simulink model "SimulinkFullblock"  (R2019b)
settings: Solver=VariableStepAuto  StartTime=0.0  StopTime=10  RelTol=1e-3
(part 1 of 5)
settings Model: Creator=gasserelazab  LastModifiedBy=gasserelazab
settings DataIOCC: ReturnWorkspaceOutputs=off
settings DebuggingCC: ArithmeticOperatorsInVariantConditions=warning
settings SFSimCC: SimUseLocalCustomCode=off  CustomCodeUndefinedFunction=UseInterfaceOnly
settings RTWCC: RTWUseLocalCustomCode=off

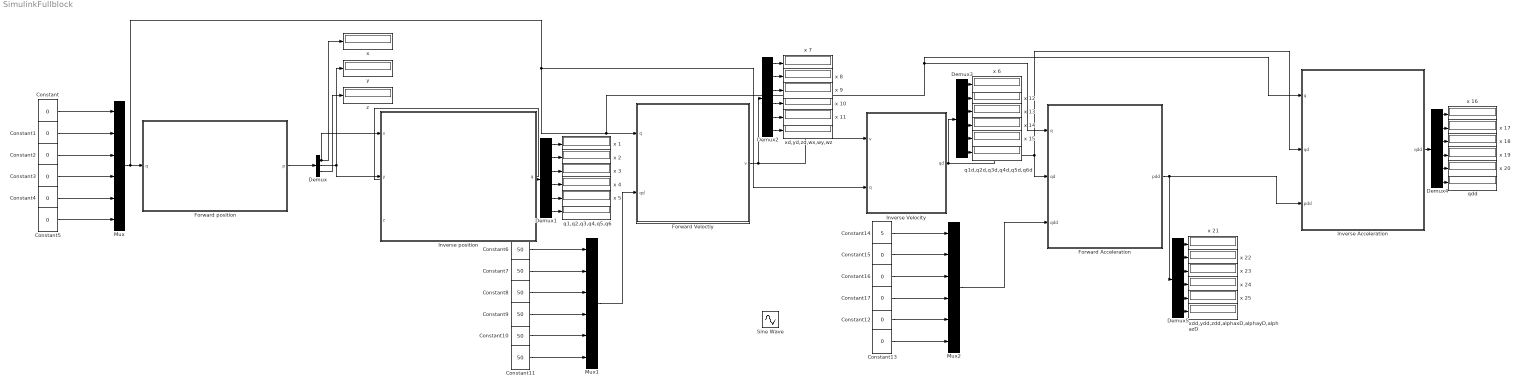
== system SimulinkFullblock ==
  " Inverse Velocity " : MATLAB Function  TreatAsAtomicUnit=on
  " xd,yd,zd,wx,wy,wz " : Display
  Constant{,1..5,12..13,15..17} (11 alike) : Constant  Value=0
  Constant{6..11} (6 alike) : Constant  Value=50
  Constant14 : Constant  Value=5
  Demux : Demux  Outputs=3
  Demux{1..5} (5 alike) : Demux  Outputs=6
  "Forward Acceleration " : MATLAB Function  TreatAsAtomicUnit=on
  Forward Veloctiy : MATLAB Function  TreatAsAtomicUnit=on
  "Forward position " : MATLAB Function  TreatAsAtomicUnit=on
  "Inverse Acceleration " : MATLAB Function  TreatAsAtomicUnit=on
  "Inverse position " : MATLAB Function  TreatAsAtomicUnit=on
  Mux : Mux  Inputs=6
  Mux1 : Mux  Inputs=6
  Mux2 : Mux  Inputs=6
  Sine Wave : Sin  SampleTime=0
  "q1,q2,q3,q4,q5,q6 " : Display
  "q1d,q2d,q3d,q4d,q5d,q6d " : Display
  "qdd " : Display
  x {,1..25} (26 alike) : Display
  "xdd,ydd,zdd,alphaxD,alphayD,alphazD " : Display
  y : Display
  z : Display
  wires:
  Mux/1 -> " Inverse Velocity "/2(q), "Inverse Acceleration "/1(q), "Forward Acceleration "/1(q), Forward Veloctiy/1(q), "Forward position "/1(q)
  Constant/1 -> Mux/1
  Constant1/1 -> Mux/2
  Constant2/1 -> Mux/3
  Constant3/1 -> Mux/4
  Constant4/1 -> Mux/5
  Constant5/1 -> Mux/6
  "Forward position "/1(p) -> Demux/1
  Demux/1 -> "Inverse position "/1(x), "x "/1
  Demux/2 -> "Inverse position "/2(y), y/1
  Demux/3 -> z/1
  "Inverse position "/1(q) -> Demux1/1
  Constant8/1 -> Mux1/3
  Constant6/1 -> Mux1/1
  Constant7/1 -> Mux1/2
  Mux1/1 -> Forward Veloctiy/2(qd)
  Constant9/1 -> Mux1/4
  Constant10/1 -> Mux1/5
  Constant11/1 -> Mux1/6
  Forward Veloctiy/1(v) -> Demux2/1, " Inverse Velocity "/1(v)
  " Inverse Velocity "/1(qd) -> Demux3/1, "Inverse Acceleration "/2(qd), "Forward Acceleration "/2(qd)
  Constant16/1 -> Mux2/3
  Constant13/1 -> Mux2/6
  Constant12/1 -> Mux2/5
  Constant15/1 -> Mux2/2
  Constant17/1 -> Mux2/4
  Mux2/1 -> "Forward Acceleration "/3(qdd)
  "Forward Acceleration "/1(pdd) -> Demux5/1, "Inverse Acceleration "/3(pdd)
  "Inverse Acceleration "/1(qdd) -> Demux4/1
  Demux1/2 -> x 2/1
  Demux1/1 -> x 1/1
  Demux1/3 -> x 3/1
  Demux1/4 -> x 4/1
  Demux1/5 -> x 5/1
  Demux1/6 -> "q1,q2,q3,q4,q5,q6 "/1
  Demux2/4 -> x 10/1
  Demux2/6 -> " xd,yd,zd,wx,wy,wz "/1
  Demux2/5 -> x 11/1
  Demux2/1 -> x 7/1
  Demux2/3 -> x 9/1
  Demux2/2 -> x 8/1
  Constant14/1 -> Mux2/1
  Demux3/5 -> x 15/1
  Demux3/4 -> x 14/1
  Demux3/6 -> "q1d,q2d,q3d,q4d,q5d,q6d "/1
  Demux3/3 -> x 13/1
  Demux3/2 -> x 12/1
  Demux3/1 -> x 6/1
  Demux4/1 -> x 16/1
  Demux4/2 -> x 17/1
  Demux4/3 -> x 18/1
  Demux4/4 -> x 19/1
  Demux4/5 -> x 20/1
  Demux4/6 -> "qdd "/1
  Demux5/6 -> "xdd,ydd,zdd,alphaxD,alphayD,alphazD "/1
  Demux5/2 -> x 22/1
  Demux5/5 -> x 25/1
  Demux5/1 -> x 21/1
  Demux5/4 -> x 24/1
  Demux5/3 -> x 23/1

== matlab function SimulinkFullblock/Inverse position  ==
  data: q output; x input; y input; z input
function q   = fcn(x, y, z)

qnew=[0;0;0;0;0;0];
qold=[50;50;50;50;50;50];

i=100;
dog=true;

while (i>0 && dog)
    q1=qold(1,1);
    q2=qold(2,1);
    q3=qold(3,1);
    q4=qold(4,1);
    q5=qold(5,1);
    q6=qold(6,1);
    
    F= [ 10*cos((pi*(q1 - 90))/180)*sin((pi*(q2 - 90))/180) - 10*sin((pi*(q5 + 90))/180)*(sin((pi*(q1 - 90))/180)*sin((pi*(q4 + 90))/180) - cos((pi*(q1 - 90))/180)*cos((pi*(q2 - 90))/180)*cos((pi*(q4 + 90))/180)) - x + cos((pi*(q1 - 90))/180)*sin((pi*(q2 - 90))/180)*(q3 + 10) - 10*cos((pi*(q1 - 90))/180)*cos((pi*(q5 + 90))/180)*sin((pi*(q2 - 90))/180);...
 10*sin((pi*(q5 + 90))/180)*(cos((pi*(q1 - 90))/180)*sin((pi*(q4 + 90))/180) + cos((pi*(q2 - 90))/180)*cos((pi*(q4 + 90))/180)*sin((pi*(q1 - 90))/180)) - y + 10*sin((pi*(q1 - 90))/180)*sin((pi*(q2 - 90))/180) + sin((pi*(q1 - 90))/180)*sin((pi*(q2 - 90))/180)*(q3 + 10) - 10*cos((pi*(q5 + 90))/180)*sin((pi*(q1 - 90))/180)*sin((pi*(q2 - 90))/180);...
                                                                                                                                                10*cos((pi*(q2 - 90))/180) - z + cos((pi*(q2 - 90))/180)*(q3 + 10) - 10*cos((pi*(q2 - 90))/180)*cos((pi*(q5 + 90))/180) - 10*cos((pi*(q4 + 90))/180)*sin((pi*(q2 - 90))/180)*sin((pi*(q5 + 90))/180) + 10];
 FJ= [ (pi*cos((pi*(q5 + 90))/180)*sin((pi*(q1 - 90))/180)*sin((pi*(q2 - 90))/180))/18 - (pi*sin((pi*(q1 - 90))/180)*sin((pi*(q2 - 90))/180))/18 - (pi*sin((pi*(q1 - 90))/180)*sin((pi*(q2 - 90))/180)*(q3 + 10))/180 - 10*sin((pi*(q5 + 90))/180)*((pi*cos((pi*(q1 - 90))/180)*sin((pi*(q4 + 90))/180))/180 + (pi*cos((pi*(q2 - 90))/180)*cos((pi*(q4 + 90))/180)*sin((pi*(q1 - 90))/180))/180), (pi*cos((pi*(q1 - 90))/180)*cos((pi*(q2 - 90))/180))/18 + (pi*cos((pi*(q1 - 90))/180)*cos((pi*(q2 - 90))/180)*(q3 + 10))/180 - (pi*cos((pi*(q1 - 90))/180)*cos((pi*(q2 - 90))/180)*cos((pi*(q5 + 90))/180))/18 - (pi*cos((pi*(q1 - 90))/180)*cos((pi*(q4 + 90))/180)*sin((pi*(q2 - 90))/180)*sin((pi*(q5 + 90))/180))/18, cos((pi*(q1 - 90))/180)*sin((pi*(q2 - 90))/180), -10*sin((pi*(q5 + 90))/180)*((pi*cos((pi*(q4 + 90))/180)*sin((pi*(q1 - 90))/180))/180 + (pi*cos((pi*(q1 - 90))/180)*cos((pi*(q2 - 90))/180)*sin((pi*(q4 + 90))/180))/180), (pi*cos((pi*(q1 - 90))/180)*sin((pi*(q2 - 90))/180)*sin((pi*(q5 + 90))/180))/18 - (pi*cos((pi*(q5 + 90))/180)*(sin((pi*(q1 - 90))/180)*sin((pi*(q4 + 90))/180) - cos((pi*(q1 - 90))/180)*cos((pi*(q2 - 90))/180)*cos((pi*(q4 + 90))/180)))/18, 0;...
 (pi*cos((pi*(q1 - 90))/180)*sin((pi*(q2 - 90))/180))/18 - 10*sin((pi*(q5 + 90))/180)*((pi*sin((pi*(q1 - 90))/180)*sin((pi*(q4 + 90))/180))/180 - (pi*cos((pi*(q1 - 90))/180)*cos((pi*(q2 - 90))/180)*cos((pi*(q4 + 90))/180))/180) + (pi*cos((pi*(q1 - 90))/180)*sin((pi*(q2 - 90))/180)*(q3 + 10))/180 - (pi*cos((pi*(q1 - 90))/180)*cos((pi*(q5 + 90))/180)*sin((pi*(q2 - 90))/180))/18, (pi*cos((pi*(q2 - 90))/180)*sin((pi*(q1 - 90))/180))/18 + (pi*cos((pi*(q2 - 90))/180)*sin((pi*(q1 - 90))/180)*(q3 + 10))/180 - (pi*cos((pi*(q2 - 90))/180)*cos((pi*(q5 + 90))/180)*sin((pi*(q1 - 90))/180))/18 - (pi*cos((pi*(q4 + 90))/180)*sin((pi*(q1 - 90))/180)*sin((pi*(q2 - 90))/180)*sin((pi*(q5 + 90))/180))/18, sin((pi*(q1 - 90))/180)*sin((pi*(q2 - 90))/180),  10*sin((pi*(q5 + 90))/180)*((pi*cos((pi*(q1 - 90))/180)*cos((pi*(q4 + 90))/180))/180 - (pi*cos((pi*(q2 - 90))/180)*sin((pi*(q1 - 90))/180)*sin((pi*(q4 + 90))/180))/180), (pi*cos((pi*(q5 + 90))/180)*(cos((pi*(q1 - 90))/180)*sin((pi*(q4 + 90))/180) + cos((pi*(q2 - 90))/180)*cos((pi*(q4 + 90))/180)*sin((pi*(q1 - 90))/180)))/18 + (pi*sin((pi*(q1 - 90))/180)*sin((pi*(q2 - 90))/180)*sin((pi*(q5 + 90))/180))/18, 0;...
                                                                                                                                                                                                                                                                                                                                                                                         0,                                                                                                 (pi*cos((pi*(q5 + 90))/180)*sin((pi*(q2 - 90))/180))/18 - (pi*sin((pi*(q2 - 90))/180)*(q3 + 10))/180 - (pi*sin((pi*(q2 - 90))/180))/18 - (pi*cos((pi*(q2 - 90))/180)*cos((pi*(q4 + 90))/180)*sin((pi*(q5 + 90))/180))/18,                         cos((pi*(q2 - 90))/180),                                                                                           (pi*sin((pi*(q2 - 90))/180)*sin((pi*(q4 + 90))/180)*sin((pi*(q5 + 90))/180))/18,                                                                                                     (pi*cos((pi*(q2 - 90))/180)*sin((pi*(q5 + 90))/180))/18 - (pi*cos((pi*(q4 + 90))/180)*cos((pi*(q5 + 90))/180)*sin((pi*(q2 - 90))/180))/18, 0];
 

    inverseFJ= transpose(FJ)*(inv(FJ*transpose(FJ)));
        
 
    qnew=qold-inverseFJ*F;
    %disp(inverseFJ*F);
    
  
   
    count=0;
   
   	for xx = 1:6
        if  ((qnew(xx,1)-qold(xx,1)<0.1) && (qnew(xx,1)-qold(xx,1)>-0.1 ))       
             count=count+1;
         end
   
    end
    
    if( count == 6)
        dog=false;
    end
    
    i=i-1;
    
    %disp(i);
    
    qold=qnew;
    
end
q=qold;

== matlab function SimulinkFullblock/Forward position  ==
  data: p output; q input
function p  = fcn(q)
q1= q(1);
q2= q(2);
q3= q(3);
q4= q(4);
q5= q(5);
q6= q(6);
L1=10;
L2=10;
L3=10;
L4=10;
pp= [ sin((pi*q6)/180)*(cos((pi*(q4 + 90))/180)*sin((pi*(q1 - 90))/180) + cos((pi*(q1 - 90))/180)*cos((pi*(q2 - 90))/180)*sin((pi*(q4 + 90))/180)) - cos((pi*q6)/180)*(cos((pi*(q5 + 90))/180)*(sin((pi*(q1 - 90))/180)*sin((pi*(q4 + 90))/180) - cos((pi*(q1 - 90))/180)*cos((pi*(q2 - 90))/180)*cos((pi*(q4 + 90))/180)) - cos((pi*(q1 - 90))/180)*sin((pi*(q2 - 90))/180)*sin((pi*(q5 + 90))/180)),   sin((pi*q6)/180)*(cos((pi*(q5 + 90))/180)*(sin((pi*(q1 - 90))/180)*sin((pi*(q4 + 90))/180) - cos((pi*(q1 - 90))/180)*cos((pi*(q2 - 90))/180)*cos((pi*(q4 + 90))/180)) - cos((pi*(q1 - 90))/180)*sin((pi*(q2 - 90))/180)*sin((pi*(q5 + 90))/180)) + cos((pi*q6)/180)*(cos((pi*(q4 + 90))/180)*sin((pi*(q1 - 90))/180) + cos((pi*(q1 - 90))/180)*cos((pi*(q2 - 90))/180)*sin((pi*(q4 + 90))/180)), - sin((pi*(q5 + 90))/180)*(sin((pi*(q1 - 90))/180)*sin((pi*(q4 + 90))/180) - cos((pi*(q1 - 90))/180)*cos((pi*(q2 - 90))/180)*cos((pi*(q4 + 90))/180)) - cos((pi*(q1 - 90))/180)*cos((pi*(q5 + 90))/180)*sin((pi*(q2 - 90))/180), cos((pi*(q1 - 90))/180)*sin((pi*(q2 - 90))/180)*(L2 + q3) - L4*(sin((pi*(q5 + 90))/180)*(sin((pi*(q1 - 90))/180)*sin((pi*(q4 + 90))/180) - cos((pi*(q1 - 90))/180)*cos((pi*(q2 - 90))/180)*cos((pi*(q4 + 90))/180)) + cos((pi*(q1 - 90))/180)*cos((pi*(q5 + 90))/180)*sin((pi*(q2 - 90))/180)) + L3*cos((pi*(q1 - 90))/180)*sin((pi*(q2 - 90))/180);
 cos((pi*q6)/180)*(cos((pi*(q5 + 90))/180)*(cos((pi*(q1 - 90))/180)*sin((pi*(q4 + 90))/180) + cos((pi*(q2 - 90))/180)*cos((pi*(q4 + 90))/180)*sin((pi*(q1 - 90))/180)) + sin((pi*(q1 - 90))/180)*sin((pi*(q2 - 90))/180)*sin((pi*(q5 + 90))/180)) - sin((pi*q6)/180)*(cos((pi*(q1 - 90))/180)*cos((pi*(q4 + 90))/180) - cos((pi*(q2 - 90))/180)*sin((pi*(q1 - 90))/180)*sin((pi*(q4 + 90))/180)), - sin((pi*q6)/180)*(cos((pi*(q5 + 90))/180)*(cos((pi*(q1 - 90))/180)*sin((pi*(q4 + 90))/180) + cos((pi*(q2 - 90))/180)*cos((pi*(q4 + 90))/180)*sin((pi*(q1 - 90))/180)) + sin((pi*(q1 - 90))/180)*sin((pi*(q2 - 90))/180)*sin((pi*(q5 + 90))/180)) - cos((pi*q6)/180)*(cos((pi*(q1 - 90))/180)*cos((pi*(q4 + 90))/180) - cos((pi*(q2 - 90))/180)*sin((pi*(q1 - 90))/180)*sin((pi*(q4 + 90))/180)),   sin((pi*(q5 + 90))/180)*(cos((pi*(q1 - 90))/180)*sin((pi*(q4 + 90))/180) + cos((pi*(q2 - 90))/180)*cos((pi*(q4 + 90))/180)*sin((pi*(q1 - 90))/180)) - cos((pi*(q5 + 90))/180)*sin((pi*(q1 - 90))/180)*sin((pi*(q2 - 90))/180), L4*(sin((pi*(q5 + 90))/180)*(cos((pi*(q1 - 90))/180)*sin((pi*(q4 + 90))/180) + cos((pi*(q2 - 90))/180)*cos((pi*(q4 + 90))/180)*sin((pi*(q1 - 90))/180)) - cos((pi*(q5 + 90))/180)*sin((pi*(q1 - 90))/180)*sin((pi*(q2 - 90))/180)) + sin((pi*(q1 - 90))/180)*sin((pi*(q2 - 90))/180)*(L2 + q3) + L3*sin((pi*(q1 - 90))/180)*sin((pi*(q2 - 90))/180);
                                                                                                                                                                                 cos((pi*q6)/180)*(cos((pi*(q2 - 90))/180)*sin((pi*(q5 + 90))/180) - cos((pi*(q4 + 90))/180)*cos((pi*(q5 + 90))/180)*sin((pi*(q2 - 90))/180)) - sin((pi*q6)/180)*sin((pi*(q2 - 90))/180)*sin((pi*(q4 + 90))/180),                                                                                                                                                                                 - sin((pi*q6)/180)*(cos((pi*(q2 - 90))/180)*sin((pi*(q5 + 90))/180) - cos((pi*(q4 + 90))/180)*cos((pi*(q5 + 90))/180)*sin((pi*(q2 - 90))/180)) - cos((pi*q6)/180)*sin((pi*(q2 - 90))/180)*sin((pi*(q4 + 90))/180),                                                                                                     - cos((pi*(q2 - 90))/180)*cos((pi*(q5 + 90))/180) - cos((pi*(q4 + 90))/180)*sin((pi*(q2 - 90))/180)*sin((pi*(q5 + 90))/180),                                                                                                                                                L1 - L4*(cos((pi*(q2 - 90))/180)*cos((pi*(q5 + 90))/180) + cos((pi*(q4 + 90))/180)*sin((pi*(q2 - 90))/180)*sin((pi*(q5 + 90))/180)) + cos((pi*(q2 - 90))/180)*(L2 + q3) + L3*cos((pi*(q2 - 90))/180);
                                                                                                                                                                                                                                                                                                                                                                                               0,                                                                                                                                                                                                                                                                                                                                                                                                 0,                                                                                                                                                                                                                               0,                                                                                                                                                                                                                                                                                                                                                   1];
x=pp(1,4);
y=pp(2,4);
z=pp(3,4);
p= [x;y;z];

== matlab function SimulinkFullblock/Forward Veloctiy ==
  data: q input; v output; qd input
function v   = fcn(q,qd)
q1= q(1);
q2= q(2);
q3= q(3);
q4= q(4);
q5= q(5);
q6= q(6);
q1d=qd(1);
q2d=qd(2);
q3d=qd(3);
q4d=qd(4);
q5d=qd(5);
q6d=qd(6);
L1=10;
L2=10;
L3=10;
L4=10;

A0T1= [ cos(0.0175*q1 - 1.5708),  0, -sin(0.0175*q1 - 1.5708),  0;...
 sin(0.0175*q1 - 1.5708),  0,  cos(0.0175*q1 - 1.5708),  0;...
                       0, -1,                        0, L1];
                   


A0T2= [ cos(0.0175*q1 - 1.5708)*cos(0.0175*q2 - 1.5708), -sin(0.0175*q1 - 1.5708), cos(0.0175*q1 - 1.5708)*sin(0.0175*q2 - 1.5708),  0;...
 cos(0.0175*q2 - 1.5708)*sin(0.0175*q1 - 1.5708),  cos(0.0175*q1 - 1.5708), sin(0.0175*q1 - 1.5708)*sin(0.0175*q2 - 1.5708),  0;...
                        -sin(0.0175*q2 - 1.5708),                        0,                         cos(0.0175*q2 - 1.5708), L1];
                                        
A0T3=  [ cos(0.0175*q1 - 1.5708)*cos(0.0175*q2 - 1.5708), -sin(0.0175*q1 - 1.5708), cos(0.0175*q1 - 1.5708)*sin(0.0175*q2 - 1.5708), cos(0.0175*q1 - 1.5708)*sin(0.0175*q2 - 1.5708)*(L2 + q3);...
 cos(0.0175*q2 - 1.5708)*sin(0.0175*q1 - 1.5708),  cos(0.0175*q1 - 1.5708), sin(0.0175*q1 - 1.5708)*sin(0.0175*q2 - 1.5708), sin(0.0175*q1 - 1.5708)*sin(0.0175*q2 - 1.5708)*(L2 + q3);...
                        -sin(0.0175*q2 - 1.5708),                        0,                         cos(0.0175*q2 - 1.5708),                    L1 + cos(0.0175*q2 - 1.5708)*(L2 + q3)];
                    
A0T4= [ cos(0.0175*q1 - 1.5708)*cos(0.0175*q2 - 1.5708)*cos(0.0175*q4 + 1.5708) - sin(0.0175*q1 - 1.5708)*sin(0.0175*q4 + 1.5708), cos(0.0175*q1 - 1.5708)*sin(0.0175*q2 - 1.5708), cos(0.0175*q4 + 1.5708)*sin(0.0175*q1 - 1.5708) + cos(0.0175*q1 - 1.5708)*cos(0.0175*q2 - 1.5708)*sin(0.0175*q4 + 1.5708), cos(0.0175*q1 - 1.5708)*sin(0.0175*q2 - 1.5708)*(L2 + q3) + L3*cos(0.0175*q1 - 1.5708)*sin(0.0175*q2 - 1.5708);...
 cos(0.0175*q1 - 1.5708)*sin(0.0175*q4 + 1.5708) + cos(0.0175*q2 - 1.5708)*cos(0.0175*q4 + 1.5708)*sin(0.0175*q1 - 1.5708), sin(0.0175*q1 - 1.5708)*sin(0.0175*q2 - 1.5708), cos(0.0175*q2 - 1.5708)*sin(0.0175*q1 - 1.5708)*sin(0.0175*q4 + 1.5708) - cos(0.0175*q1 - 1.5708)*cos(0.0175*q4 + 1.5708), sin(0.0175*q1 - 1.5708)*sin(0.0175*q2 - 1.5708)*(L2 + q3) + L3*sin(0.0175*q1 - 1.5708)*sin(0.0175*q2 - 1.5708);...
                                                                          -cos(0.0175*q4 + 1.5708)*sin(0.0175*q2 - 1.5708),                         cos(0.0175*q2 - 1.5708),                                                                          -sin(0.0175*q2 - 1.5708)*sin(0.0175*q4 + 1.5708),                                            L1 + cos(0.0175*q2 - 1.5708)*(L2 + q3) + L3*cos(0.0175*q2 - 1.5708)];
                                                                      
A0T5= [ cos(0.0175*q1 - 1.5708)*sin(0.0175*q2 - 1.5708)*sin(0.0175*q5 + 1.5708) - cos(0.0175*q5 + 1.5708)*(sin(0.0175*q1 - 1.5708)*sin(0.0175*q4 + 1.5708) - cos(0.0175*q1 - 1.5708)*cos(0.0175*q2 - 1.5708)*cos(0.0175*q4 + 1.5708)), cos(0.0175*q4 + 1.5708)*sin(0.0175*q1 - 1.5708) + cos(0.0175*q1 - 1.5708)*cos(0.0175*q2 - 1.5708)*sin(0.0175*q4 + 1.5708), - sin(0.0175*q5 + 1.5708)*(sin(0.0175*q1 - 1.5708)*sin(0.0175*q4 + 1.5708) - cos(0.0175*q1 - 1.5708)*cos(0.0175*q2 - 1.5708)*cos(0.0175*q4 + 1.5708)) - cos(0.0175*q1 - 1.5708)*cos(0.0175*q5 + 1.5708)*sin(0.0175*q2 - 1.5708), cos(0.0175*q1 - 1.5708)*sin(0.0175*q2 - 1.5708)*(L2 + q3) + L3*cos(0.0175*q1 - 1.5708)*sin(0.0175*q2 - 1.5708);...
 cos(0.0175*q5 + 1.5708)*(cos(0.0175*q1 - 1.5708)*sin(0.0175*q4 + 1.5708) + cos(0.0175*q2 - 1.5708)*cos(0.0175*q4 + 1.5708)*sin(0.0175*q1 - 1.5708)) + sin(0.0175*q1 - 1.5708)*sin(0.0175*q2 - 1.5708)*sin(0.0175*q5 + 1.5708), cos(0.0175*q2 - 1.5708)*sin(0.0175*q1 - 1.5708)*sin(0.0175*q4 + 1.5708) - cos(0.0175*q1 - 1.5708)*cos(0.0175*q4 + 1.5708),   sin(0.0175*q5 + 1.5708)*(cos(0.0175*q1 - 1.5708)*sin(0.0175*q4 + 1.5708) + cos(0.0175*q2 - 1.5708)*cos(0.0175*q4 + 1.5708)*sin(0.0175*q1 - 1.5708)) - cos(0.0175*q5 + 1.5708)*sin(0.0175*q1 - 1.5708)*sin(0.0175*q2 - 1.5708), sin(0.0175*q1 - 1.5708)*sin(0.0175*q2 - 1.5708)*(L2 + q3) + L3*sin(0.0175*q1 - 1.5708)*sin(0.0175*q2 - 1.5708);...
                                                                                                     cos(0.0175*q2 - 1.5708)*sin(0.0175*q5 + 1.5708) - cos(0.0175*q4 + 1.5708)*cos(0.0175*q5 + 1.5708)*sin(0.0175*q2 - 1.5708),                                                                          -sin(0.0175*q2 - 1.5708)*sin(0.0175*q4 + 1.5708),                                                                                                     - cos(0.0175*q2 - 1.5708)*cos(0.0175*q5 + 1.5708) - cos(0.0175*q4 + 1.5708)*sin(0.0175*q2 - 1.5708)*sin(0.0175*q5 + 1.5708),                                            L1 + cos(0.0175*q2 - 1.5708)*(L2 + q3) + L3*cos(0.0175*q2 - 1.5708)];
                                                                                                 
                                                                                                 
A0T6= [ sin((pi*q6)/180)*(cos((pi*(q4 + 90))/180)*sin((pi*(q1 - 90))/180) + cos((pi*(q1 - 90))/180)*cos((pi*(q2 - 90))/180)*sin((pi*(q4 + 90))/180)) - cos((pi*q6)/180)*(cos((pi*(q5 + 90))/180)*(sin((pi*(q1 - 90))/180)*sin((pi*(q4 + 90))/180) - cos((pi*(q1 - 90))/180)*cos((pi*(q2 - 90))/180)*cos((pi*(q4 + 90))/180)) - cos((pi*(q1 - 90))/180)*sin((pi*(q2 - 90))/180)*sin((pi*(q5 + 90))/180)),   sin((pi*q6)/180)*(cos((pi*(q5 + 90))/180)*(sin((pi*(q1 - 90))/180)*sin((pi*(q4 + 90))/180) - cos((pi*(q1 - 90))/180)*cos((pi*(q2 - 90))/180)*cos((pi*(q4 + 90))/180)) - cos((pi*(q1 - 90))/180)*sin((pi*(q2 - 90))/180)*sin((pi*(q5 + 90))/180)) + cos((pi*q6)/180)*(cos((pi*(q4 + 90))/180)*sin((pi*(q1 - 90))/180) + cos((pi*(q1 - 90))/180)*cos((pi*(q2 - 90))/180)*sin((pi*(q4 + 90))/180)), - sin((pi*(q5 + 90))/180)*(sin((pi*(q1 - 90))/180)*sin((pi*(q4 + 90))/180) - cos((pi*(q1 - 90))/180)*cos((pi*(q2 - 90))/180)*cos((pi*(q4 + 90))/180)) - cos((pi*(q1 - 90))/180)*cos((pi*(q5 + 90))/180)*sin((pi*(q2 - 90))/180), cos((pi*(q1 - 90))/180)*sin((pi*(q2 - 90))/180)*(L2 + q3) - L4*(sin((pi*(q5 + 90))/180)*(sin((pi*(q1 - 90))/180)*sin((pi*(q4 + 90))/180) - cos((pi*(q1 - 90))/180)*cos((pi*(q2 - 90))/180)*cos((pi*(q4 + 90))/180)) + cos((pi*(q1 - 90))/180)*cos((pi*(q5 + 90))/180)*sin((pi*(q2 - 90))/180)) + L3*cos((pi*(q1 - 90))/180)*sin((pi*(q2 - 90))/180);
 cos((pi*q6)/180)*(cos((pi*(q5 + 90))/180)*(cos((pi*(q1 - 90))/180)*sin((pi*(q4 + 90))/180) + cos((pi*(q2 - 90))/180)*cos((pi*(q4 + 90))/180)*sin((pi*(q1 - 90))/180)) + sin((pi*(q1 - 90))/180)*sin((pi*(q2 - 90))/180)*sin((pi*(q5 + 90))/180)) - sin((pi*q6)/180)*(cos((pi*(q1 - 90))/180)*cos((pi*(q4 + 90))/180) - cos((pi*(q2 - 90))/180)*sin((pi*(q1 - 90))/180)*sin((pi*(q4 + 90))/180)), - sin((pi*q6)/180)*(cos((pi*(q5 + 90))/180)*(cos((pi*(q1 - 90))/180)*sin((pi*(q4 + 90))/180) + cos((pi*(q2 - 90))/180)*cos((pi*(q4 + 90))/180)*sin((pi*(q1 - 90))/180)) + sin((pi*(q1 - 90))/180)*sin((pi*(q2 - 90))/180)*sin((pi*(q5 + 90))/180)) - cos((pi*q6)/180)*(cos((pi*(q1 - 90))/180)*cos((pi*(q4 + 90))/180) - cos((pi*(q2 - 90))/180)*sin((pi*(q1 - 90))/180)*sin((pi*(q4 + 90))/180)),   sin((pi*(q5 + 90))/180)*(cos((pi*(q1 - 90))/180)*sin((pi*(q4 + 90))/180) + cos((pi*(q2 - 90))/180)*cos((pi*(q4 + 90))/180)*sin((pi*(q1 - 90))/180)) - cos((pi*(q5 + 90))/180)*sin((pi*(q1 - 90))/180)*sin((pi*(q2 - 90))/180), L4*(sin((pi*(q5 + 90))/180)*(cos((pi*(q1 - 90))/180)*sin((pi*(q4 + 90))/180) + cos((pi*(q2 - 90))/180)*cos((pi*(q4 + 90))/180)*sin((pi*(q1 - 90))/180)) - cos((pi*(q5 + 90))/180)*sin((pi*(q1 - 90))/180)*sin((pi*(q2 - 90))/180)) + sin((pi*(q1 - 90))/180)*sin((pi*(q2 - 90))/180)*(L2 + q3) + L3*sin((pi*(q1 - 90))/180)*sin((pi*(q2 - 90))/180);
                                                                                                                                                                                 cos((pi*q6)/180)*(cos((pi*(q2 - 90))/180)*sin((pi*(q5 + 90))/180) - cos((pi*(q4 + 90))/180)*cos((pi*(q5 + 90))/180)*sin((pi*(q2 - 90))/180)) - sin((pi*q6)/180)*sin((pi*(q2 - 90))/180)*sin((pi*(q4 + 90))/180),                                                                                                                                                                                 - sin((pi*q6)/180)*(cos((pi*(q2 - 90))/180)*sin((pi*(q5 + 90))/180) - cos((pi*(q4 + 90))/180)*cos((pi*(q5 + 90))/180)*sin((pi*(q2 - 90))/180)) - cos((pi*q6)/180)*sin((pi*(q2 - 90))/180)*sin((pi*(q4 + 90))/180),                                                                                                     - cos((pi*(q2 - 90))/180)*cos((pi*(q5 + 90))/180) - cos((pi*(q4 + 90))/180)*sin((pi*(q2 - 90))/180)*sin((pi*(q5 + 90))/180),                                                                                                                                                L1 - L4*(cos((pi*(q2 - 90))/180)*cos((pi*(q5 + 90))/180) + cos((pi*(q4 + 90))/180)*sin((pi*(q2 - 90))/180)*sin((pi*(q5 + 90))/180)) + cos((pi*(q2 - 90))/180)*(L2 + q3) + L3*cos((pi*(q2 - 90))/180)];
                                                                                                                                                                                                                                  
                                                                                                                   
 
Jv1= cross([0;0;1], A0T6(:,4)-[0;0;0]); 
Jv2= cross(A0T1(:,3),(A0T6(:,4)-A0T1(:,4)));
Jv3= A0T3(:,3);
Jv4= cross(A0T3(:,3),(A0T6(:,4)-A0T3(:,4)));
Jv5= cross(A0T4(:,3),(A0T6(:,4)-A0T4(:,4)));
Jv6= cross(A0T5(:,3),(A0T6(:,4)-A0T5(:,4)));

Jw1=[0;0;1];
Jw2= A0T1(:,3);
Jw3=[0;0;0];
Jw4= A0T3(:,3);
Jw5= A0T4(:,3);
Jw6= A0T5(:,3);
v= [Jv1 Jv2 Jv3 Jv4 Jv5 Jv6; Jw1 Jw2 Jw3 Jw4 Jw5 Jw6]*[q1d;q2d;q3d;q4d;q5d;q6d];

== matlab function SimulinkFullblock/ Inverse Velocity  ==
  data: v input; qd output; q input
function qd  = fcn(v,q)
xd=v(1);
yd=v(2);
zd=v(3);
wx=v(4);
wy=v(5);
wz=v(6);
q1= q(1);
q2= q(2);
q3= q(3);
q4= q(4);
q5= q(5);
q6= q(6);
L1=10;
L2=10;
L3=10;
L4=10;

A0T1= [ cos(0.0175*q1 - 1.5708),  0, -sin(0.0175*q1 - 1.5708),  0;...
 sin(0.0175*q1 - 1.5708),  0,  cos(0.0175*q1 - 1.5708),  0;...
                       0, -1,                        0, L1];
                   


A0T2= [ cos(0.0175*q1 - 1.5708)*cos(0.0175*q2 - 1.5708), -sin(0.0175*q1 - 1.5708), cos(0.0175*q1 - 1.5708)*sin(0.0175*q2 - 1.5708),  0;...
 cos(0.0175*q2 - 1.5708)*sin(0.0175*q1 - 1.5708),  cos(0.0175*q1 - 1.5708), sin(0.0175*q1 - 1.5708)*sin(0.0175*q2 - 1.5708),  0;...
                        -sin(0.0175*q2 - 1.5708),                        0,                         cos(0.0175*q2 - 1.5708), L1];
                                        
A0T3=  [ cos(0.0175*q1 - 1.5708)*cos(0.0175*q2 - 1.5708), -sin(0.0175*q1 - 1.5708), cos(0.0175*q1 - 1.5708)*sin(0.0175*q2 - 1.5708), cos(0.0175*q1 - 1.5708)*sin(0.0175*q2 - 1.5708)*(L2 + q3);...
 cos(0.0175*q2 - 1.5708)*sin(0.0175*q1 - 1.5708),  cos(0.0175*q1 - 1.5708), sin(0.0175*q1 - 1.5708)*sin(0.0175*q2 - 1.5708), sin(0.0175*q1 - 1.5708)*sin(0.0175*q2 - 1.5708)*(L2 + q3);...
                        -sin(0.0175*q2 - 1.5708),                        0,                         cos(0.0175*q2 - 1.5708),                    L1 + cos(0.0175*q2 - 1.5708)*(L2 + q3)];
                    
A0T4= [ cos(0.0175*q1 - 1.5708)*cos(0.0175*q2 - 1.5708)*cos(0.0175*q4 + 1.5708) - sin(0.0175*q1 - 1.5708)*sin(0.0175*q4 + 1.5708), cos(0.0175*q1 - 1.5708)*sin(0.0175*q2 - 1.5708), cos(0.0175*q4 + 1.5708)*sin(0.0175*q1 - 1.5708) + cos(0.0175*q1 - 1.5708)*cos(0.0175*q2 - 1.5708)*sin(0.0175*q4 + 1.5708), cos(0.0175*q1 - 1.5708)*sin(0.0175*q2 - 1.5708)*(L2 + q3) + L3*cos(0.0175*q1 - 1.5708)*sin(0.0175*q2 - 1.5708);...
 cos(0.0175*q1 - 1.5708)*sin(0.0175*q4 + 1.5708) + cos(0.0175*q2 - 1.5708)*cos(0.0175*q4 + 1.5708)*sin(0.0175*q1 - 1.5708), sin(0.0175*q1 - 1.5708)*sin(0.0175*q2 - 1.5708), cos(0.0175*q2 - 1.5708)*sin(0.0175*q1 - 1.5708)*sin(0.0175*q4 + 1.5708) - cos(0.0175*q1 - 1.5708)*cos(0.0175*q4 + 1.5708), sin(0.0175*q1 - 1.5708)*sin(0.0175*q2 - 1.5708)*(L2 + q3) + L3*sin(0.0175*q1 - 1.5708)*sin(0.0175*q2 - 1.5708);...
                                                                          -cos(0.0175*q4 + 1.5708)*sin(0.0175*q2 - 1.5708),                         cos(0.0175*q2 - 1.5708),                                                                          -sin(0.0175*q2 - 1.5708)*sin(0.0175*q4 + 1.5708),                                            L1 + cos(0.0175*q2 - 1.5708)*(L2 + q3) + L3*cos(0.0175*q2 - 1.5708)];
                                                                      
A0T5= [ cos(0.0175*q1 - 1.5708)*sin(0.0175*q2 - 1.5708)*sin(0.0175*q5 + 1.5708) - cos(0.0175*q5 + 1.5708)*(sin(0.0175*q1 - 1.5708)*sin(0.0175*q4 + 1.5708) - cos(0.0175*q1 - 1.5708)*cos(0.0175*q2 - 1.5708)*cos(0.0175*q4 + 1.5708)), cos(0.0175*q4 + 1.5708)*sin(0.0175*q1 - 1.5708) + cos(0.0175*q1 - 1.5708)*cos(0.0175*q2 - 1.5708)*sin(0.0175*q4 + 1.5708), - sin(0.0175*q5 + 1.5708)*(sin(0.0175*q1 - 1.5708)*sin(0.0175*q4 + 1.5708) - cos(0.0175*q1 - 1.5708)*cos(0.0175*q2 - 1.5708)*cos(0.0175*q4 + 1.5708)) - cos(0.0175*q1 - 1.5708)*cos(0.0175*q5 + 1.5708)*sin(0.0175*q2 - 1.5708), cos(0.0175*q1 - 1.5708)*sin(0.0175*q2 - 1.5708)*(L2 + q3) + L3*cos(0.0175*q1 - 1.5708)*sin(0.0175*q2 - 1.5708);...
 cos(0.0175*q5 + 1.5708)*(cos(0.0175*q1 - 1.5708)*sin(0.0175*q4 + 1.5708) + cos(0.0175*q2 - 1.5708)*cos(0.0175*q4 + 1.5708)*sin(0.0175*q1 - 1.5708)) + sin(0.0175*q1 - 1.5708)*sin(0.0175*q2 - 1.5708)*sin(0.0175*q5 + 1.5708), cos(0.0175*q2 - 1.5708)*sin(0.0175*q1 - 1.5708)*sin(0.0175*q4 + 1.5708) - cos(0.0175*q1 - 1.5708)*cos(0.0175*q4 + 1.5708),   sin(0.0175*q5 + 1.5708)*(cos(0.0175*q1 - 1.5708)*sin(0.0175*q4 + 1.5708) + cos(0.0175*q2 - 1.5708)*cos(0.0175*q4 + 1.5708)*sin(0.0175*q1 - 1.5708)) - cos(0.0175*q5 + 1.5708)*sin(0.0175*q1 - 1.5708)*sin(0.0175*q2 - 1.5708), sin(0.0175*q1 - 1.5708)*sin(0.0175*q2 - 1.5708)*(L2 + q3) + L3*sin(0.0175*q1 - 1.5708)*sin(0.0175*q2 - 1.5708);...
                                                                                                     cos(0.0175*q2 - 1.5708)*sin(0.0175*q5 + 1.5708) - cos(0.0175*q4 + 1.5708)*cos(0.0175*q5 + 1.5708)*sin(0.0175*q2 - 1.5708),                                                                          -sin(0.0175*q2 - 1.5708)*sin(0.0175*q4 + 1.5708),                                                                                                     - cos(0.0175*q2 - 1.5708)*cos(0.0175*q5 + 1.5708) - cos(0.0175*q4 + 1.5708)*sin(0.0175*q2 - 1.5708)*sin(0.0175*q5 + 1.5708),                                            L1 + cos(0.0175*q2 - 1.5708)*(L2 + q3) + L3*cos(0.0175*q2 - 1.5708)];
                                                                                                 
                                                                                                 
A0T6= [ sin((pi*q6)/180)*(cos((pi*(q4 + 90))/180)*sin((pi*(q1 - 90))/180) + cos((pi*(q1 - 90))/180)*cos((pi*(q2 - 90))/180)*sin((pi*(q4 + 90))/180)) - cos((pi*q6)/180)*(cos((pi*(q5 + 90))/180)*(sin((pi*(q1 - 90))/180)*sin((pi*(q4 + 90))/180) - cos((pi*(q1 - 90))/180)*cos((pi*(q2 - 90))/180)*cos((pi*(q4 + 90))/180)) - cos((pi*(q1 - 90))/180)*sin((pi*(q2 - 90))/180)*sin((pi*(q5 + 90))/180)),   sin((pi*q6)/180)*(cos((pi*(q5 + 90))/180)*(sin((pi*(q1 - 90))/180)*sin((pi*(q4 + 90))/180) - cos((pi*(q1 - 90))/180)*cos((pi*(q2 - 90))/180)*cos((pi*(q4 + 90))/180)) - cos((pi*(q1 - 90))/180)*sin((pi*(q2 - 90))/180)*sin((pi*(q5 + 90))/180)) + cos((pi*q6)/180)*(cos((pi*(q4 + 90))/180)*sin((pi*(q1 - 90))/180) + cos((pi*(q1 - 90))/180)*cos((pi*(q2 - 90))/180)*sin((pi*(q4 + 90))/180)), - sin((pi*(q5 + 90))/180)*(sin((pi*(q1 - 90))/180)*sin((pi*(q4 + 90))/180) - cos((pi*(q1 - 90))/180)*cos((pi*(q2 - 90))/180)*cos((pi*(q4 + 90))/180)) - cos((pi*(q1 - 90))/180)*cos((pi*(q5 + 90))/180)*sin((pi*(q2 - 90))/180), cos((pi*(q1 - 90))/180)*sin((pi*(q2 - 90))/180)*(L2 + q3) - L4*(sin((pi*(q5 + 90))/180)*(sin((pi*(q1 - 90))/180)*sin((pi*(q4 + 90))/180) - cos((pi*(q1 - 90))/180)*cos((pi*(q2 - 90))/180)*cos((pi*(q4 + 90))/180)) + cos((pi*(q1 - 90))/180)*cos((pi*(q5 + 90))/180)*sin((pi*(q2 - 90))/180)) + L3*cos((pi*(q1 - 90))/180)*sin((pi*(q2 - 90))/180);
 cos((pi*q6)/180)*(cos((pi*(q5 + 90))/180)*(cos((pi*(q1 - 90))/180)*sin((pi*(q4 + 90))/180) + cos((pi*(q2 - 90))/180)*cos((pi*(q4 + 90))/180)*sin((pi*(q1 - 90))/180)) + sin((pi*(q1 - 90))/180)*sin((pi*(q2 - 90))/180)*sin((pi*(q5 + 90))/180)) - sin((pi*q6)/180)*(cos((pi*(q1 - 90))/180)*cos((pi*(q4 + 90))/180) - cos((pi*(q2 - 90))/180)*sin((pi*(q1 - 90))/180)*sin((pi*(q4 + 90))/180)), - sin((pi*q6)/180)*(cos((pi*(q5 + 90))/180)*(cos((pi*(q1 - 90))/180)*sin((pi*(q4 + 90))/180) + cos((pi*(q2 - 90))/180)*cos((pi*(q4 + 90))/180)*sin((pi*(q1 - 90))/180)) + sin((pi*(q1 - 90))/180)*sin((pi*(q2 - 90))/180)*sin((pi*(q5 + 90))/180)) - cos((pi*q6)/180)*(cos((pi*(q1 - 90))/180)*cos((pi*(q4 + 90))/180) - cos((pi*(q2 - 90))/180)*sin((pi*(q1 - 90))/180)*sin((pi*(q4 + 90))/180)),   sin((pi*(q5 + 90))/180)*(cos((pi*(q1 - 90))/180)*sin((pi*(q4 + 90))/180) + cos((pi*(q2 - 90))/180)*cos((pi*(q4 + 90))/180)*sin((pi*(q1 - 90))/180)) - cos((pi*(q5 + 90))/180)*sin((pi*(q1 - 90))/180)*sin((pi*(q2 - 90))/180), L4*(sin((pi*(q5 + 90))/180)*(cos((pi*(q1 - 90))/180)*sin((pi*(q4 + 90))/180) + cos((pi*(q2 - 90))/180)*cos((pi*(q4 + 90))/180)*sin((pi*(q1 - 90))/180)) - cos((pi*(q5 + 90))/180)*sin((pi*(q1 - 90))/180)*sin((pi*(q2 - 90))/180)) + sin((pi*(q1 - 90))/180)*sin((pi*(q2 - 90))/180)*(L2 + q3) + L3*sin((pi*(q1 - 90))/180)*sin((pi*(q2 - 90))/180);
                                                                                                                                                                                 cos((pi*q6)/180)*(cos((pi*(q2 - 90))/180)*sin((pi*(q5 + 90))/180) - cos((pi*(q4 + 90))/180)*cos((pi*(q5 + 90))/180)*sin((pi*(q2 - 90))/180)) - sin((pi*q6)/180)*sin((pi*(q2 - 90))/180)*sin((pi*(q4 + 90))/180),                                                                                                                                                                                 - sin((pi*q6)/180)*(cos((pi*(q2 - 90))/180)*sin((pi*(q5 + 90))/180) - cos((pi*(q4 + 90))/180)*cos((pi*(q5 + 90))/180)*sin((pi*(q2 - 90))/180)) - cos((pi*q6)/180)*sin((pi*(q2 - 90))/180)*sin((pi*(q4 + 90))/180),                                                                                                     - cos((pi*(q2 - 90))/180)*cos((pi*(q5 + 90))/180) - cos((pi*(q4 + 90))/180)*sin((pi*(q2 - 90))/180)*sin((pi*(q5 + 90))/180),                                                                                                                                                L1 - L4*(cos((pi*(q2 - 90))/180)*cos((pi*(q5 + 90))/180) + cos((pi*(q4 + 90))/180)*sin((pi*(q2 - 90))/180)*sin((pi*(q5 + 90))/180)) + cos((pi*(q2 - 90))/180)*(L2 + q3) + L3*cos((pi*(q2 - 90))/180)];
                                                                                                                                                                                                                                  
                                                                                                                   
 
Jv1= cross([0;0;1], A0T6(:,4)-[0;0;0]); 
Jv2= cross(A0T1(:,3),(A0T6(:,4)-A0T1(:,4)));
Jv3= A0T3(:,3);
Jv4= cross(A0T3(:,3),(A0T6(:,4)-A0T3(:,4)));
Jv5= cross(A0T4(:,3),(A0T6(:,4)-A0T4(:,4)));
Jv6= cross(A0T5(:,3),(A0T6(:,4)-A0T5(:,4)));

Jw1=[0;0;1];
Jw2= A0T1(:,3);
Jw3=[0;0;0];
Jw4= A0T3(:,3);
Jw5= A0T4(:,3);
Jw6= A0T5(:,3);
VelocityMat= [Jv1 Jv2 Jv3 Jv4 Jv5 Jv6; Jw1 Jw2 Jw3 Jw4 Jw5 Jw6];
inverseVMAT= transpose(VelocityMat)*(inv(VelocityMat*transpose(VelocityMat)));
qd= inverseVMAT*[xd;yd;zd;wx;wy;wz];
